simulink subsystem "main_CA"  (R2025a)
settings: Solver=VariableStepAuto  StartTime=0.0  StopTime=10.0  RelTol=1e-3
undefined symbols (not defined in the file or in its folder): vehicle
settings Model: Creator=gurt1  LastModifiedBy=gurt1

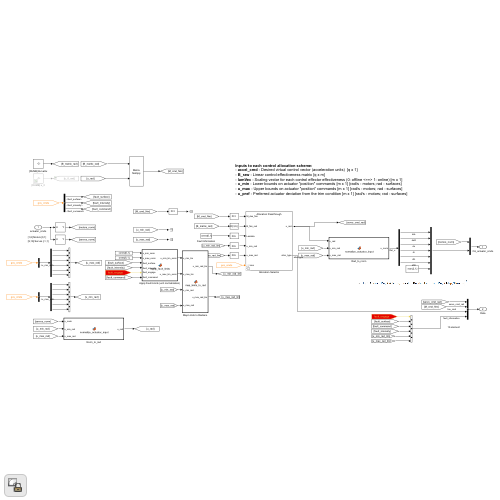
[thumbnail: Simulink's stored preview of the top-level diagram]
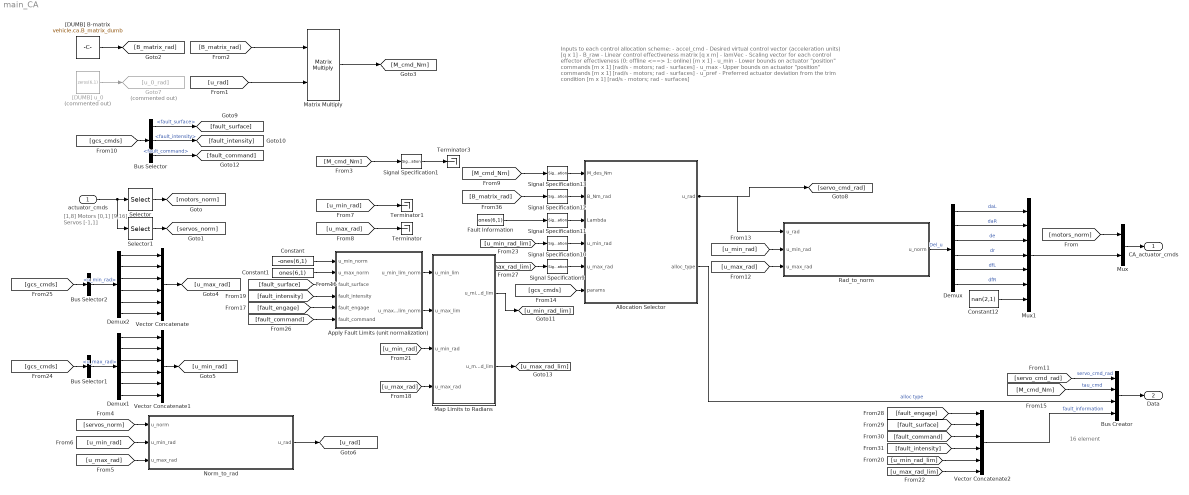
== system main_CA ==
  note: 16 element
  note: [1,8] Motors [0,1]
      | [9,16] Servos [-1,1]
  note: Inputs to each control allocation scheme:
      | - accel_cmd - Desired virtual control vector (acceleration units) [q x 1]
      | - B_raw - Linear control effectiveness matrix [q x m]
      | - lamVec - Scaling vector for each control effector effectiveness (0: offline <==> 1: online) [m x 1]
      | - u_min - Lower bounds on actuator "position" commands [m x 1] [rad/s - motors; rad - surfaces]
      | - u_max - Upper bounds on actuator "position" commands [m x 1] [rad/s - motors; rad - surfaces]
      | - u_pref - Preferred actuator deviation from the trim condition [m x 1] [rad/s - motors; rad - surfaces]
  actuator_cmds : Inport
  Allocation Selector : Subsystem  Variant=on  EmptyChoice=on
  Apply Fault Limits (unit normalization) : MATLAB Function  TreatAsAtomicUnit=on
  Bus Creator : BusCreator  Inputs=4
  Bus Selector : BusSelector  OutputSignals=Fault.fault_surface,Fault.fault_intensity,Fault.fault_command
  Bus Selector1 : BusSelector  OutputSignals=ca.u_max_rad
  Bus Selector2 : BusSelector  OutputSignals=ca.u_min_rad
  Constant : Constant  Value=-ones(6,1)
  Constant1 : Constant  Value=ones(6,1)
  Constant12 : Constant  Value=nan(2,1)
  Demux : Demux  Outputs=6
  Demux1 : Demux  Outputs=6
  Demux2 : Demux  Outputs=6
  Fault Information : Constant  Value=ones(6,1)
  Goto7 : Goto  Commented=on  GotoTag=u_0_rad
  Map Limits to Radians : MATLAB Function  TreatAsAtomicUnit=on
  Matrix Multiply : Product  Multiplication=Matrix(*)
  Mux : Mux  Inputs=2
  Mux1 : Mux  Inputs=7
  Norm_to_rad : MATLAB Function  TreatAsAtomicUnit=on
  Rad_to_norm : MATLAB Function  TreatAsAtomicUnit=on
  Selector : Selector  InputPortWidth=16  IndexOptions=Index vector (dialog)  Indices=[1:8]  OutputSizes=1
  Selector1 : Selector  InputPortWidth=16  IndexOptions=Index vector (dialog)  Indices=[9:14]  OutputSizes=1
  Signal Specification1 : SignalSpecification  Dimensions=3
  Signal Specification10 : SignalSpecification  Dimensions=6
  Signal Specification11 : SignalSpecification  Dimensions=6
  Signal Specification12 : SignalSpecification  Dimensions=[3,6]
  Signal Specification13 : SignalSpecification  Dimensions=3
  Signal Specification9 : SignalSpecification  Dimensions=6
  Terminator : Terminator
  Terminator1 : Terminator
  Terminator3 : Terminator
  Vector Concatenate : Concatenate  NumInputs=6
  Vector Concatenate1 : Concatenate  NumInputs=6
  Vector Concatenate2 : Concatenate  NumInputs=6
  "[DUMB] B-matrix" : Constant  Value=vehicle.ca.B_matrix_dumb
  "[DUMB] u_0" : Constant  Commented=on  Value=zeros(6,1)
  CA_actuator_cmds : Outport
  Data : Outport  Port=2
  wires:
  actuator_cmds/1 -> Selector/1, Selector1/1
  Selector/1 -> [motors_norm]
  Selector1/1 -> [servos_norm]
  Mux/1 -> CA_actuator_cmds/1
  [motors_norm] -> Mux/1
  [B_matrix_rad] -> Matrix Multiply/1
  [u_rad] -> Matrix Multiply/2
  "[DUMB] B-matrix"/1 -> [B_matrix_rad]
  Matrix Multiply/1 -> [M_cmd_Nm]
  Demux2/1 -> Vector Concatenate/1
  Demux2/2 -> Vector Concatenate/2
  Demux2/3 -> Vector Concatenate/3
  Demux2/4 -> Vector Concatenate/4
  Demux2/5 -> Vector Concatenate/5
  Demux2/6 -> Vector Concatenate/6
  Vector Concatenate/1 -> [u_max_rad]
  Vector Concatenate1/1 -> [u_min_rad]
  Demux1/6 -> Vector Concatenate1/6
  Demux1/5 -> Vector Concatenate1/5
  Demux1/4 -> Vector Concatenate1/4
  Demux1/3 -> Vector Concatenate1/3
  Demux1/2 -> Vector Concatenate1/2
  Demux1/1 -> Vector Concatenate1/1
  Constant12/1 -> Mux1/7
  Mux1/1 -> Mux/2
  [u_max_rad] -> Norm_to_rad/3(u_max_rad)
  [servos_norm] -> Norm_to_rad/1(u_norm)
  [u_min_rad] -> Norm_to_rad/2(u_min_rad)
  [u_max_rad] -> Terminator/1
  [u_min_rad] -> Terminator1/1
  Norm_to_rad/1(u_rad) -> [u_rad]
  [M_cmd_Nm] -> Signal Specification1/1
  [B_matrix_rad] -> Signal Specification12/1
  [M_cmd_Nm] -> Signal Specification13/1
  Fault Information/1 -> Signal Specification11/1
  Signal Specification1/1 -> Terminator3/1
  Rad_to_norm/1(u_norm) -> Demux/1  "Del_u"
  [u_min_rad] -> Rad_to_norm/2(u_min_rad)
  [u_max_rad] -> Rad_to_norm/3(u_max_rad)
  Demux/1 -> Mux1/1  "daL"
  Demux/2 -> Mux1/2  "daR"
  Demux/3 -> Mux1/3  "de"
  Demux/4 -> Mux1/4  "dr"
  Demux/5 -> Mux1/5  "dfL"
  Demux/6 -> Mux1/6  "dfR"
  "[DUMB] u_0"/1 -> Goto7/1
  Constant/1 -> Apply Fault Limits (unit normalization)/1(u_min_norm)
  Constant1/1 -> Apply Fault Limits (unit normalization)/2(u_max_norm)
  [gcs_cmds] -> Bus Selector/1
  Apply Fault Limits (unit normalization)/1(u_min_lim_norm) -> Map Limits to Radians/1(u_min_lim)
  Apply Fault Limits (unit normalization)/2(u_max_lim_norm) -> Map Limits to Radians/2(u_max_lim)
  Bus Creator/1 -> Data/1
  [servo_cmd_rad] -> Bus Creator/1  "servo_cmd_rad"
  [M_cmd_Nm] -> Bus Creator/2  "tau_cmd"
  Bus Selector/1 -> [fault_surface]  "<fault_surface>"
  Bus Selector/2 -> [fault_intensity]  "<fault_intensity>"
  [fault_surface] -> Apply Fault Limits (unit normalization)/3(fault_surface)
  [fault_engage] -> Apply Fault Limits (unit normalization)/5(fault_engage)
  [fault_intensity] -> Apply Fault Limits (unit normalization)/4(fault_intensity)
  [gcs_cmds] -> Bus Selector1/1
  [gcs_cmds] -> Bus Selector2/1
  Bus Selector1/1 -> Demux1/1  "<u_max_rad>"
  Bus Selector2/1 -> Demux2/1  "<u_min_rad>"
  Bus Selector/3 -> [fault_command]  "<fault_command>"
  [fault_command] -> Apply Fault Limits (unit normalization)/6(fault_command)
  [u_min_rad] -> Map Limits to Radians/3(u_min_rad)
  [u_max_rad] -> Map Limits to Radians/4(u_max_rad)
  Map Limits to Radians/1(u_min_rad_lim) -> [u_min_rad_lim]
  Map Limits to Radians/2(u_max_rad_lim) -> [u_max_rad_lim]
  [u_min_rad_lim] -> Signal Specification10/1
  [u_max_rad_lim] -> Signal Specification9/1
  [fault_engage] -> Vector Concatenate2/1
  [fault_surface] -> Vector Concatenate2/2
  [fault_command] -> Vector Concatenate2/3
  [fault_intensity] -> Vector Concatenate2/4
  [u_min_rad_lim] -> Vector Concatenate2/5
  [u_max_rad_lim] -> Vector Concatenate2/6
  Vector Concatenate2/1 -> Bus Creator/4  "fault_information"
  Signal Specification13/1 -> Allocation Selector/1(M_des_Nm)
  Signal Specification12/1 -> Allocation Selector/2(B_Nm_rad)
  Signal Specification11/1 -> Allocation Selector/3(Lambda)
  Signal Specification10/1 -> Allocation Selector/4(u_min_rad)
  Signal Specification9/1 -> Allocation Selector/5(u_max_rad)
  [gcs_cmds] -> Allocation Selector/6(params)
  Allocation Selector/1(u_rad) -> Rad_to_norm/1(u_rad), [servo_cmd_rad]
  Allocation Selector/2(alloc_type) -> Bus Creator/3  "alloc type"

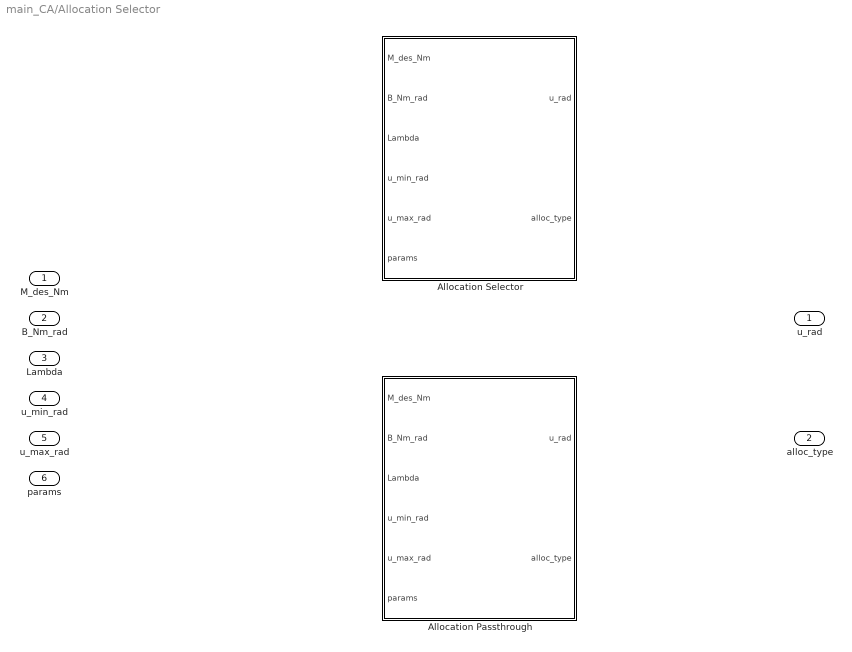
== system main_CA/Allocation Selector ==
  M_des_Nm : Inport
  B_Nm_rad : Inport  Port=2
  Lambda : Inport  Port=3
  u_min_rad : Inport  Port=4
  u_max_rad : Inport  Port=5
  params : Inport  Port=6
  Allocation Passthrough : Subsystem  VariantControl=enable_alloc == 0
  Allocation Selector : Subsystem  VariantControl=enable_alloc == 1
  u_rad : Outport
  alloc_type : Outport  Port=2

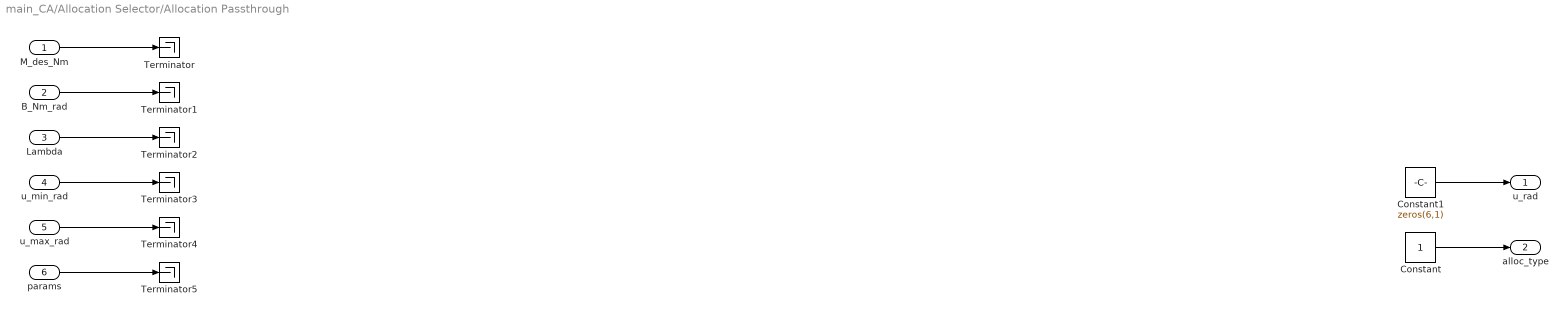
== system main_CA/Allocation Selector/Allocation Passthrough ==
  M_des_Nm : Inport
  B_Nm_rad : Inport  Port=2
  Lambda : Inport  Port=3
  u_min_rad : Inport  Port=4
  u_max_rad : Inport  Port=5
  params : Inport  Port=6
  Constant : Constant
  Constant1 : Constant  Value=zeros(6,1)
  Terminator{,1..5} (6 alike) : Terminator
  u_rad : Outport
  alloc_type : Outport  Port=2
  wires:
  M_des_Nm/1 -> Terminator/1
  B_Nm_rad/1 -> Terminator1/1
  Lambda/1 -> Terminator2/1
  u_min_rad/1 -> Terminator3/1
  u_max_rad/1 -> Terminator4/1
  params/1 -> Terminator5/1
  Constant1/1 -> u_rad/1
  Constant/1 -> alloc_type/1

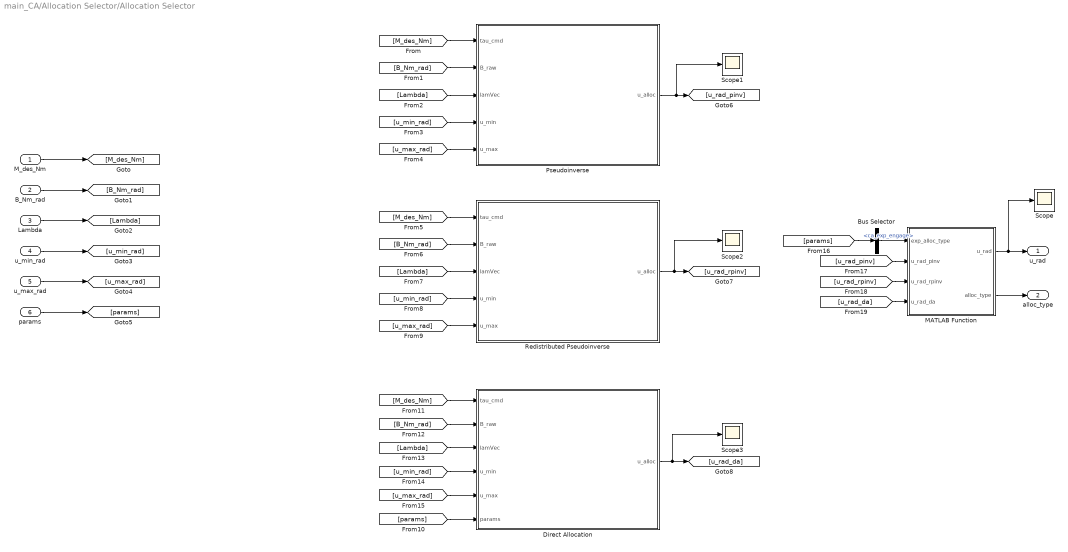
== system main_CA/Allocation Selector/Allocation Selector ==
  M_des_Nm : Inport
  B_Nm_rad : Inport  Port=2
  Lambda : Inport  Port=3
  u_min_rad : Inport  Port=4
  u_max_rad : Inport  Port=5
  params : Inport  Port=6
  Bus Selector : BusSelector  OutputSignals=Fault.ca_exp_engage
  Direct Allocation : Subsystem
  MATLAB Function : MATLAB Function  TreatAsAtomicUnit=on
  Pseudoinverse : Subsystem
  Redistributed Pseudoinverse : Subsystem
  Scope{,1..3} (4 alike) : Scope
      Scope settings: ActiveDisplayYMinimum=-0.65449846949787349  ActiveDisplayYMaximum=0.65449846949787349  DataLoggingVariableName=ScopeData2
      Scope1 settings: ActiveDisplayYMinimum=-0.35537218474428556  ActiveDisplayYMaximum=0.64346909028762467  DataLoggingVariableName=ScopeData3
      Scope2 settings: ActiveDisplayYMinimum=-0.46134886884172194  ActiveDisplayYMaximum=0.63303740275830112  DataLoggingVariableName=ScopeData5
      Scope3 settings: DataLoggingVariableName=ScopeData6
  u_rad : Outport
  alloc_type : Outport  Port=2
  wires:
  MATLAB Function/2(alloc_type) -> alloc_type/1
  Bus Selector/1 -> MATLAB Function/1(exp_alloc_type)  "<ca_exp_engage>"
  [u_rad_da] -> MATLAB Function/4(u_rad_da)
  [u_rad_rpinv] -> MATLAB Function/3(u_rad_rpinv)
  [u_rad_pinv] -> MATLAB Function/2(u_rad_pinv)
  MATLAB Function/1(u_rad) -> Scope/1, u_rad/1
  Direct Allocation/1(u_alloc) -> [u_rad_da], Scope3/1
  Redistributed Pseudoinverse/1(u_alloc) -> [u_rad_rpinv], Scope2/1
  Pseudoinverse/1(u_alloc) -> [u_rad_pinv], Scope1/1
  [params] -> Bus Selector/1
  [M_des_Nm] -> Direct Allocation/1(tau_cmd)
  [B_Nm_rad] -> Direct Allocation/2(B_raw)
  [Lambda] -> Direct Allocation/3(lamVec)
  [u_min_rad] -> Direct Allocation/4(u_min)
  [u_max_rad] -> Direct Allocation/5(u_max)
  [params] -> Direct Allocation/6(params)
  params/1 -> [params]
  [u_max_rad] -> Redistributed Pseudoinverse/5(u_max)
  [u_min_rad] -> Redistributed Pseudoinverse/4(u_min)
  [Lambda] -> Redistributed Pseudoinverse/3(lamVec)
  [B_Nm_rad] -> Redistributed Pseudoinverse/2(B_raw)
  [M_des_Nm] -> Redistributed Pseudoinverse/1(tau_cmd)
  [u_max_rad] -> Pseudoinverse/5(u_max)
  [u_min_rad] -> Pseudoinverse/4(u_min)
  [Lambda] -> Pseudoinverse/3(lamVec)
  [B_Nm_rad] -> Pseudoinverse/2(B_raw)
  [M_des_Nm] -> Pseudoinverse/1(tau_cmd)
  u_max_rad/1 -> [u_max_rad]
  u_min_rad/1 -> [u_min_rad]
  Lambda/1 -> [Lambda]
  B_Nm_rad/1 -> [B_Nm_rad]
  M_des_Nm/1 -> [M_des_Nm]

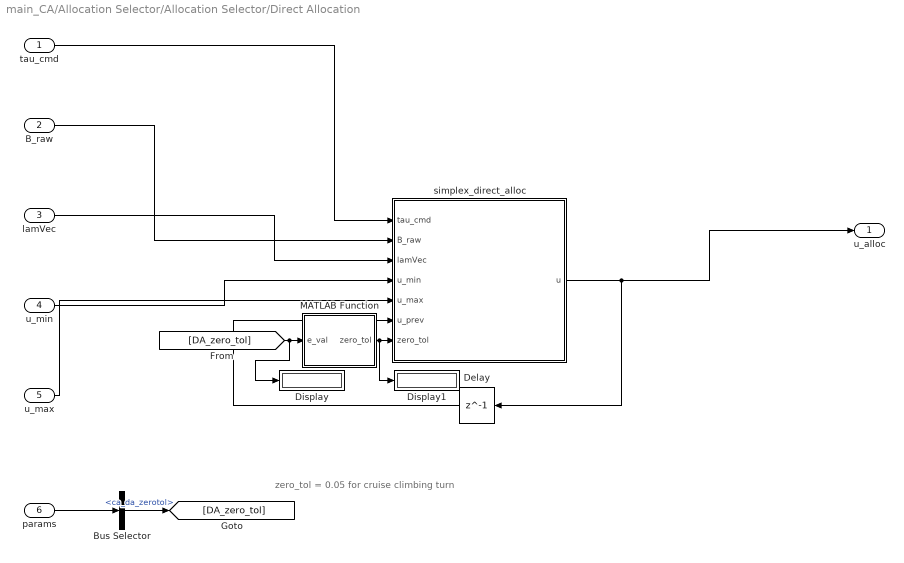
== system main_CA/Allocation Selector/Allocation Selector/Direct Allocation ==
  note: zero_tol = 0.05 for cruise climbing turn
  tau_cmd : Inport
  B_raw : Inport  Port=2
  lamVec : Inport  Port=3
  u_min : Inport  Port=4
  u_max : Inport  Port=5
  params : Inport  Port=6
  Bus Selector : BusSelector  OutputSignals=Fault.ca_da_zerotol
  Delay : Delay  DelayLength=1  InitialCondition=zeros(6,1)
  Display : Display
  Display1 : Display
  MATLAB Function : MATLAB Function  TreatAsAtomicUnit=on
  simplex_direct_alloc : MATLAB Function  TreatAsAtomicUnit=on
  u_alloc : Outport
  wires:
  MATLAB Function/1(zero_tol) -> simplex_direct_alloc/7(zero_tol), Display1/1
  params/1 -> Bus Selector/1
  Bus Selector/1 -> [DA_zero_tol]  "<ca_da_zerotol>"
  B_raw/1 -> simplex_direct_alloc/2(B_raw)
  [DA_zero_tol] -> MATLAB Function/1(e_val), Display/1
  lamVec/1 -> simplex_direct_alloc/3(lamVec)
  u_min/1 -> simplex_direct_alloc/4(u_min)
  simplex_direct_alloc/1(u) -> u_alloc/1, Delay/1
  u_max/1 -> simplex_direct_alloc/5(u_max)
  Delay/1 -> simplex_direct_alloc/6(u_prev)
  tau_cmd/1 -> simplex_direct_alloc/1(tau_cmd)

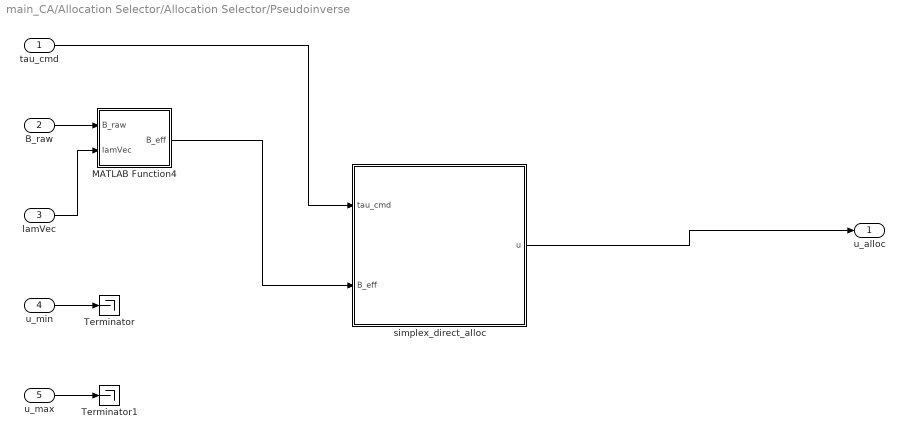
== system main_CA/Allocation Selector/Allocation Selector/Pseudoinverse ==
  tau_cmd : Inport
  B_raw : Inport  Port=2
  lamVec : Inport  Port=3
  u_min : Inport  Port=4
  u_max : Inport  Port=5
  MATLAB Function4 : MATLAB Function  TreatAsAtomicUnit=on
  Terminator : Terminator
  Terminator1 : Terminator
  simplex_direct_alloc : MATLAB Function  TreatAsAtomicUnit=on
  u_alloc : Outport
  wires:
  B_raw/1 -> MATLAB Function4/1(B_raw)
  simplex_direct_alloc/1(u) -> u_alloc/1
  u_min/1 -> Terminator/1
  u_max/1 -> Terminator1/1
  MATLAB Function4/1(B_eff) -> simplex_direct_alloc/2(B_eff)
  lamVec/1 -> MATLAB Function4/2(lamVec)
  tau_cmd/1 -> simplex_direct_alloc/1(tau_cmd)

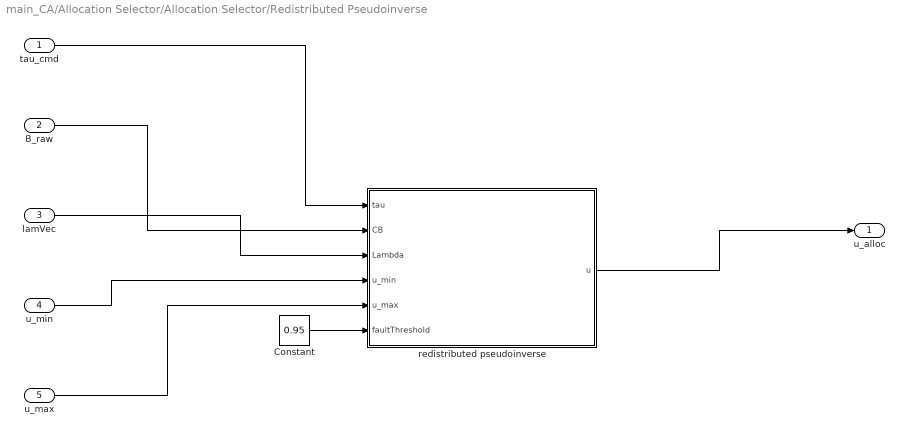
== system main_CA/Allocation Selector/Allocation Selector/Redistributed Pseudoinverse ==
  tau_cmd : Inport
  B_raw : Inport  Port=2
  lamVec : Inport  Port=3
  u_min : Inport  Port=4
  u_max : Inport  Port=5
  Constant : Constant  Value=0.95
  redistributed pseudoinverse : MATLAB Function  TreatAsAtomicUnit=on
  u_alloc : Outport
  wires:
  u_min/1 -> redistributed pseudoinverse/4(u_min)
  lamVec/1 -> redistributed pseudoinverse/3(Lambda)
  redistributed pseudoinverse/1(u) -> u_alloc/1
  u_max/1 -> redistributed pseudoinverse/5(u_max)
  B_raw/1 -> redistributed pseudoinverse/2(CB)
  tau_cmd/1 -> redistributed pseudoinverse/1(tau)
  Constant/1 -> redistributed pseudoinverse/6(faultThreshold)

== matlab function main_CA/Map Limits to Radians ==
  data: u_min_lim input double; u_min_rad_lim output double; u_max_lim input double; u_min_rad input double; u_max_rad input double; u_max_rad_lim output double
function [u_min_rad_lim, u_max_rad_lim] = map_limits_to_rad( ...
    u_min_lim, u_max_lim, u_min_rad, u_max_rad)

[u_min_rad_lim, u_max_rad_lim] = map_limits_to_rad( ...
    u_min_lim, u_max_lim, u_min_rad, u_max_rad);

== matlab function main_CA/Allocation Selector/Allocation Selector/Direct Allocation/simplex_direct_alloc ==
  data: tau_cmd input; u output; B_raw input; lamVec input; u_min input; u_max input; u_prev input; zero_tol input
function u = simplex_direct_alloc(tau_cmd, B_raw, lamVec, u_min, u_max, u_prev, zero_tol)
u = simplex_direct_alloc(tau_cmd, B_raw, lamVec, u_min, u_max, u_prev, zero_tol);

== matlab function main_CA/Allocation Selector/Allocation Selector/MATLAB Function ==
  data: exp_alloc_type input; u_rad output; u_rad_pinv input; u_rad_rpinv input; u_rad_da input; alloc_type output
function [u_rad,alloc_type] = fcn(exp_alloc_type, u_rad_pinv, u_rad_rpinv, u_rad_da)

% Traditional Pseudoinverse
if exp_alloc_type == 1
    u_rad = u_rad_pinv;
    alloc_type = 1;
% Redistributed Pseudoinverse
elseif exp_alloc_type == 2
    u_rad = u_rad_rpinv;
    alloc_type = 2;
% Direct Allocation
elseif exp_alloc_type == 3
    u_rad = u_rad_da;
    alloc_type = 3;
% Invalid Type -> zeros(6,1);
else
    u_rad = zeros(6,1);
    alloc_type = 0;
end

== matlab function main_CA/Allocation Selector/Allocation Selector/Pseudoinverse/simplex_direct_alloc ==
  data: tau_cmd input; u output; B_eff input
function u = traditional_pseudo_inverse(tau_cmd, B_eff)

u = traditional_pseudo_inverse(tau_cmd, B_eff);

== matlab function main_CA/Apply Fault Limits (unit normalization) ==
  data: u_min_norm input; u_min_lim_norm output; u_max_norm input; fault_surface input; fault_intensity input; fault_engage input; u_max_lim_norm output; fault_command input
function [u_min_lim_norm, u_max_lim_norm] = apply_fault_limits( ...
    u_min_norm, u_max_norm, fault_surface, fault_intensity, fault_engage, fault_command)

[u_min_lim_norm, u_max_lim_norm] = apply_fault_limits( ...
    u_min_norm, u_max_norm, fault_surface, fault_intensity, fault_engage, fault_command);

== matlab function main_CA/Norm_to_rad ==
  data: u_norm input; u_rad output; u_min_rad input; u_max_rad input
%% normalize_actuator_input
% DESCRIPTION: 
%   Maps normalized input [-1,1] to actuator deflection in radians using
%   element-wise limits from u_min_rad and u_max_rad.
%
% INPUTS: 
%   u_norm     - Normalized actuator input [-1,1]
%   u_min_rad  - Vector of minimum actuator limits [rad]
%   u_max_rad  - Vector of maximum actuator limits [rad]
%
% OUTPUTS:
%   u_rad      - Scaled actuator output [rad]
%
% WRITTEN BY:
%   Garrett D. Asper
%   Virginia Tech
%   Email: garrettasper@vt.edu
%
% HISTORY:
%   2025-08-25 - Created and debugged, GDA
%
% NOMENCLATURE:                                  UNITS:
%   Not Applicable                                  Not Applicable.

function u_rad = normalize_actuator_input(u_norm,u_min_rad,u_max_rad)

% Ensure same size
% if ~isequal(size(u_norm),size(u_min_rad),size(u_max_rad))
%     error('u_norm, u_min_rad, and u_max_rad must have the same size');
% end

% Linear mapping
u_rad = 0.5*((u_max_rad - u_min_rad).*u_norm + (u_max_rad + u_min_rad));

end

== matlab function main_CA/Rad_to_norm ==
  data: u_rad input; u_norm output; u_min_rad input; u_max_rad input
%% normalize_actuator_input
% DESCRIPTION: 
%   Maps actuator deflection in radians to normalized input [-1,1] using
%   element-wise limits from u_min_rad and u_max_rad.
%
% INPUTS: 
%   u_rad      - Actuator input [rad]
%   u_min_rad  - Vector of minimum actuator limits [rad]
%   u_max_rad  - Vector of maximum actuator limits [rad]
%
% OUTPUTS:
%   u_norm     - Normalized actuator output [-1,1]
%
% WRITTEN BY:
%   Garrett D. Asper
%   Virginia Tech
%   Email: garrettasper@vt.edu
%
% HISTORY:
%   2025-08-26 - Created and debugged, GDA
%
% NOMENCLATURE:                                  UNITS:
%   Not Applicable                                  Not Applicable.

function u_norm = normalize_actuator_input(u_rad,u_min_rad,u_max_rad)

% Ensure same size
% if ~isequal(size(u_rad),size(u_min_rad),size(u_max_rad))
%     error('u_rad, u_min_rad, and u_max_rad must have the same size');
% end

% Linear normalization: map [u_min,u_max] -> [-1,1]
u_norm = 2*(u_rad - u_min_rad)./(u_max_rad - u_min_rad) - 1;

end

== matlab function main_CA/Allocation Selector/Allocation Selector/Direct Allocation/MATLAB Function ==
  data: e_val input; zero_tol output
function zero_tol  = fcn(e_val)


% take the input and make it into 1*10^(e_val)
zero_tol = 1*10^(e_val);

== matlab function main_CA/Allocation Selector/Allocation Selector/Redistributed Pseudoinverse/redistributed pseudoinverse ==
  data: tau input; u output; CB input; Lambda input; u_min input; u_max input; faultThreshold input
function u = redistributed_pseudo_inverse(tau, CB, Lambda, u_min, u_max, faultThreshold)

u = redistributed_pseudo_inverse(tau, CB, Lambda, u_min, u_max, faultThreshold);

== matlab function main_CA/Allocation Selector/Allocation Selector/Pseudoinverse/MATLAB Function4 ==
  data: B_eff output; B_raw input; lamVec input
function B_eff = fcn(B_raw, lamVec)

B_eff = B_raw*diag(lamVec);
